simulink model "test_randomization"  (R2018a)
settings: Solver=VariableStepAuto  StartTime=0.0  StopTime=10.0  RelTol=1e-3
settings Model: Creator=Arsalan  LastModifiedBy=Arsalan

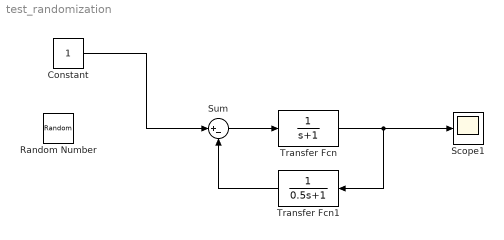
== system test_randomization ==
  Constant : Constant
  Random Number : RandomNumber  SampleTime=0.1
  Scope1 : Scope
  Sum : Sum  Inputs=|+-
  Transfer Fcn : TransferFcn  Denominator=[1 1]
  Transfer Fcn1 : TransferFcn  Denominator=[0.5 1]
  wires:
  Sum/1 -> Transfer Fcn/1
  Transfer Fcn/1 -> Transfer Fcn1/1, Scope1/1
  Transfer Fcn1/1 -> Sum/2
  Constant/1 -> Sum/1
